simulink model "sine_igntegrate"  (R2020a)
settings: Solver=VariableStepAuto  StartTime=0.0  StopTime=10.0  RelTol=1e-3
settings Model: Creator=Ganesh  LastModifiedBy=Ganesh

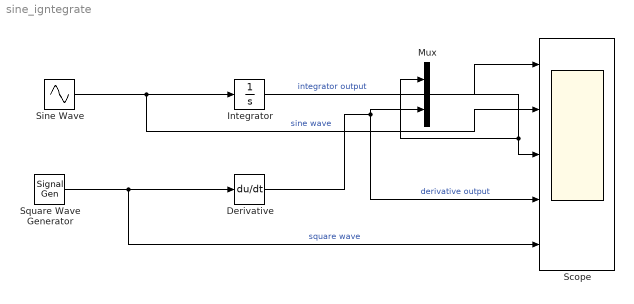
== system sine_igntegrate ==
  Derivative : Derivative
  Integrator : Integrator  InitialCondition=5
  Mux : Mux  Inputs=2
  Scope : Scope  NumInputPorts=5
  Sine Wave : Sin  Amplitude=20  SampleTime=0
  Square Wave Generator : SignalGenerator  WaveForm=square  Amplitude=20  Units=rad/sec
  wires:
  Sine Wave/1 -> Scope/2, Integrator/1  "sine wave"
  Integrator/1 -> Mux/1, Scope/3  "integrator output"
  Mux/1 -> Scope/1
  Square Wave Generator/1 -> Scope/5, Derivative/1  "square wave"
  Derivative/1 -> Scope/4, Mux/2  "derivative output"
